simulink model "Assignment3"  (R2020a)
settings: Solver=VariableStepAuto  StartTime=0.0  StopTime=10.0  RelTol=1e-3
model workspace (MAT data in the model file):
  A = 1
  Cd = 1
  Cr = 1
  I = 1
  KD = 1
  KI = 1
  KP = 4
  MD = 2
  Rho = 1
  T = 1
  Vr = 100
  Zheta = 0.261799387799
  alpha_n = 1
  d = 1
  g = 9.81
  m = 1000
settings Model: OrderedModelArguments=off  Creator=Pongsakorn  LastModifiedBy=Pongsakorn

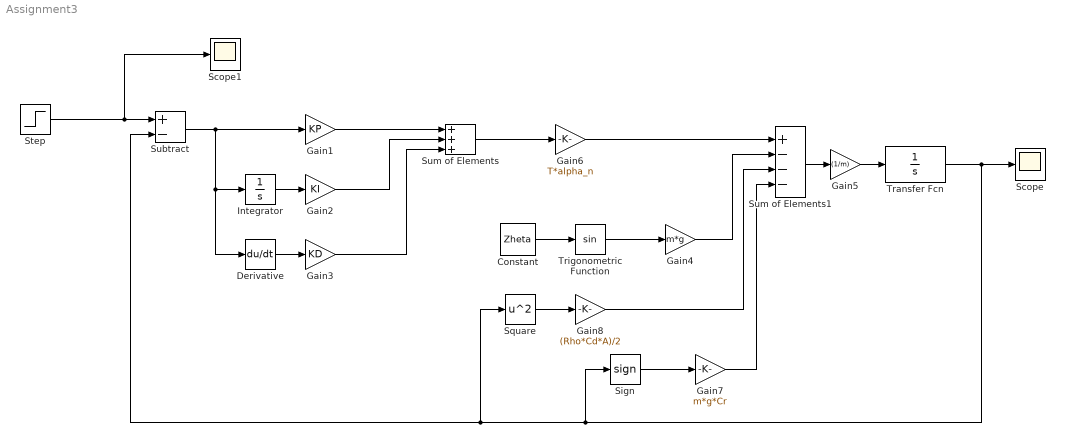
== system Assignment3 ==
  Constant : Constant  Value=Zheta
  Derivative : Derivative
  Gain1 : Gain  Gain=KP
  Gain2 : Gain  Gain=KI
  Gain3 : Gain  Gain=KD
  Gain4 : Gain  Gain=m*g
  Gain5 : Gain  Gain=(1/m)
  Gain6 : Gain  Gain=T*alpha_n
  Gain7 : Gain  Gain=m*g*Cr
  Gain8 : Gain  Gain=(Rho*Cd*A)/2
  Integrator : Integrator
  Scope : Scope
  Scope1 : Scope
  Sign : Signum  ZeroCross=off
  Square : Math  Operator=square  SaturateOnIntegerOverflow=on
  Step : Step  After=Vr  SampleTime=0
  Subtract : Sum  Inputs=+-
  Sum of Elements : Sum  Inputs=+++  CollapseMode=Specified dimension  CollapseDim=3
  Sum of Elements1 : Sum  Inputs=+---  CollapseMode=Specified dimension  CollapseDim=3
  Transfer Fcn : TransferFcn  Denominator=[1 0]
  Trigonometric Function : Trigonometry
  wires:
  Subtract/1 -> Derivative/1, Integrator/1, Gain1/1
  Integrator/1 -> Gain2/1
  Derivative/1 -> Gain3/1
  Gain1/1 -> Sum of Elements/1
  Sum of Elements1/1 -> Gain5/1
  Transfer Fcn/1 -> Sign/1, Square/1, Subtract/2, Scope/1
  Sum of Elements/1 -> Gain6/1
  Sign/1 -> Gain7/1
  Square/1 -> Gain8/1
  Trigonometric Function/1 -> Gain4/1
  Gain6/1 -> Sum of Elements1/1
  Gain5/1 -> Transfer Fcn/1
  Gain4/1 -> Sum of Elements1/2
  Constant/1 -> Trigonometric Function/1
  Gain8/1 -> Sum of Elements1/3
  Gain7/1 -> Sum of Elements1/4
  Gain2/1 -> Sum of Elements/2
  Gain3/1 -> Sum of Elements/3
  Step/1 -> Subtract/1, Scope1/1
